simulink model "Elevator_stateflow"  (R2024b)
settings: Solver=VariableStepAuto  StartTime=0.0  StopTime=inf  RelTol=1e-3
settings Model: Creator=kanith kumar  LastModifiedBy=kanith kumar

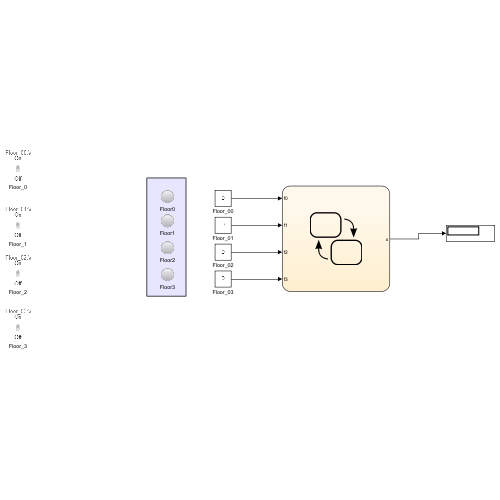
[thumbnail: Simulink's stored preview of the top-level diagram]
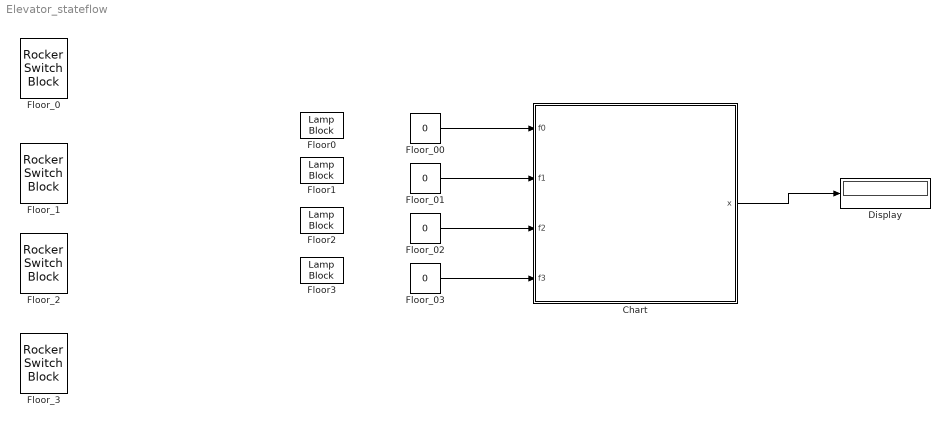
== system Elevator_stateflow ==
  Chart : Stateflow chart  TreatAsAtomicUnit=on
  Display : Display
  Floor{0..3} (4 alike) : LampBlock  LabelPosition=Hide
  Floor_{0..3} (4 alike) : RockerSwitchBlock
      settings: Values={{'Off', 'On'}, [0 1]}
  Floor_00 : Constant  Value=0
  Floor_01 : Constant  Value=0
  Floor_02 : Constant  Value=0
  Floor_03 : Constant  Value=0
  wires:
  Chart/1(x) -> Display/1
  Floor_00/1 -> Chart/1(f0)
  Floor_01/1 -> Chart/2(f1)
  Floor_02/1 -> Chart/3(f2)
  Floor_03/1 -> Chart/4(f3)

== stateflow chart Elevator_stateflow/Chart ==
  state Floor_0
    entry:
    x=0;
    state open_0
      dr_open=1
    state close_0
      dr_open=0
    (default) -> close_0
    close_0 -> open_0 : [x==0]
    open_0 -> close_0 : [x~=0]
  state Floor_1
    entry:
    x=1;
    state open_1
      dr_open=1
    state close_1
      dr_open=0
    (default) -> Floor_1.close_1
    Floor_1.close_1 -> Floor_1.open_1 : [x==1]
    Floor_1.open_1 -> Floor_1.close_1 : [x~=1]
  state Floor_2
    entry:
    x=2;
    state open_1
      dr_open=1
    state close_1
      dr_open=0
    (default) -> Floor_2.close_1
    Floor_2.close_1 -> Floor_2.open_1 : [x==2]
    Floor_2.open_1 -> Floor_2.close_1 : [x~=2]
  state Floor_3
    entry:
    x=3;
    state open_1
      dr_open=1
    state close_1
      dr_open=0
    (default) -> Floor_3.close_1
    Floor_3.close_1 -> Floor_3.open_1 : [x==3]
    Floor_3.open_1 -> Floor_3.close_1 : [x~=3]
  Floor_0 -> Floor_3 [order 3] : [f3==1]
  Floor_1 -> Floor_3 [order 2] : [f3==1]
  (default) -> Floor_0
  Floor_0 -> Floor_1 [order 1] : [f1==1]
  Floor_1 -> Floor_2 [order 1] : [f2==1]
  Floor_2 -> Floor_3 [order 1] : [f3==1]
  Floor_2 -> Floor_0 [order 2] : [f0==1]
  Floor_3 -> Floor_0 [order 3] : [f0==1]
  Floor_1 -> Floor_0 [order 3] : [f0==1]
  Floor_0 -> Floor_2 [order 2] : [f2==1]
  Floor_2 -> Floor_1 [order 3] : [f1==1]
  Floor_3 -> Floor_1 [order 2] : [f1==1]
  Floor_3 -> Floor_2 [order 1] : [f2==1]
  data: x output; dr_open local; f0 input; f1 input; f2 input; f3 input
